simulink model "closedLoopServo"  (R2019b)
settings: Solver=VariableStepAuto  StartTime=0.0  StopTime=5  FixedStep=0.002  RelTol=1e-3  EnableMultiTasking=on
undefined symbols (not defined in the file or in its folder): K0
libraries: cstblocks x2
settings Model: ExtModeTrigDuration=10000  Creator=icpmoles  LastModifiedBy=icpmoles
settings SolverCC: PositivePriorityOrder=on
settings DataIOCC: ReturnWorkspaceOutputs=off
settings OptimizationCC: LifeSpan=inf
settings DebuggingCC: ArithmeticOperatorsInVariantConditions=warning
settings SFSimCC: SimUseLocalCustomCode=off  CustomCodeUndefinedFunction=UseInterfaceOnly
settings RTWCC: Description=QUARC Win64 Target  SystemTargetFile=quarc_win64.tlc  TemplateMakefile=quarc_default_tmf  RTWUseLocalCustomCode=off
settings CodeAppCC: StateflowObjectComments=on
settings STFCustomTargetCC: TargetPreCompLibLocation=C:\PROGRA~3\QUARC\lib\2016a\win64\release  TargetLangStandard=C99 (ISO)  ConcurrentExecutionCompliant=on  GRTInterface=on  SystemTargetFile=quarc_win64.tlc
settings GRTTargetCC: TargetPreCompLibLocation=C:\PROGRA~3\QUARC\lib\2016a\win64\release  ParMdlRefBuildCompliant=off  CompOptLevelCompliant=off  CombineOutputUpdateFcns=off  MatFileLogging=off  CPPClassGenCompliant=off  GRTInterface=on  UseToolchainInfoCompliant=off  ExtMode=on  ExtModeMexFile=quarc_comm
settings ConfigComp: CovMetricSettings=dswe

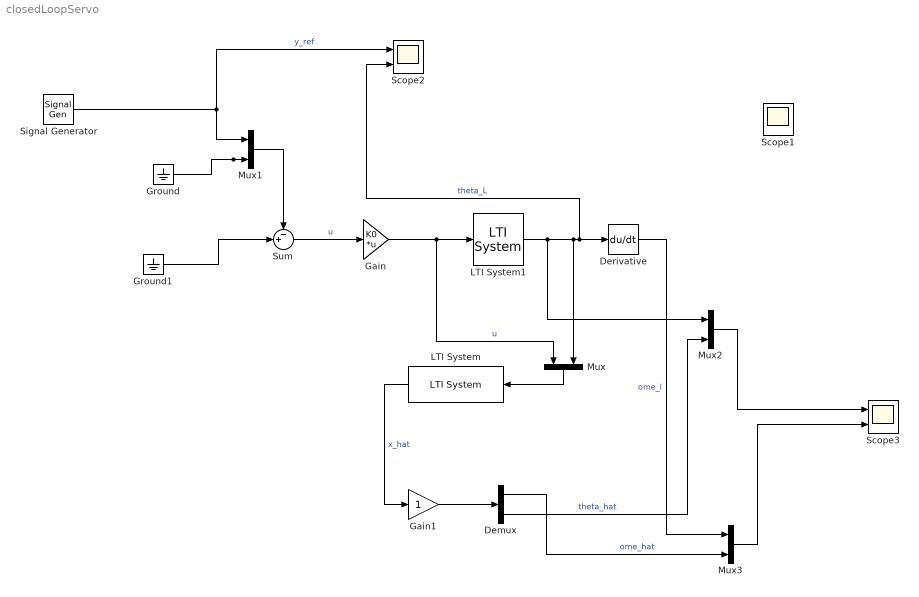
== system closedLoopServo ==
  Demux : Demux  Outputs=2
  Derivative : Derivative  CoefficientInTFapproximation=100
  Gain : Gain  Gain=K0  Multiplication=Matrix(K*u)
  Gain1 : Gain
  Ground : Ground
  Ground1 : Ground
  LTI System : cstblocks/LTI System  sys=sysObserver0  IC=[]
  LTI System1 : cstblocks/LTI System  sys=g  IC=[]
  Mux{,1..3} (4 alike) : Mux  Inputs=2
  Scope1 : Scope  NumInputPorts=3
  Scope2 : Scope  NumInputPorts=2
  Scope3 : Scope  NumInputPorts=2
  Signal Generator : SignalGenerator  WaveForm=square  Amplitude=2  Frequency=2  Units=rad/sec
  Sum : Sum  Inputs=-+|
  wires:
  LTI System1/1 -> Mux2/1, Derivative/1, Scope2/2, Mux/2  "theta_L"
  Mux/1 -> LTI System/1
  Sum/1 -> Gain/1  "u"
  Signal Generator/1 -> Scope2/1, Mux1/1  "y_ref"
  Mux1/1 -> Sum/1
  Ground/1 -> Mux1/2
  Gain/1 -> Mux/1, LTI System1/1  "u"
  Ground1/1 -> Sum/2
  Mux3/1 -> Scope3/2
  Mux2/1 -> Scope3/1
  LTI System/1 -> Gain1/1  "x_hat"
  Demux/2 -> Mux2/2  "theta_hat"
  Derivative/1 -> Mux3/1  "ome_l"
  Demux/1 -> Mux3/2  "ome_hat"
  Gain1/1 -> Demux/1
